simulink model "model2022b"  (R2022b)
settings: Solver=FixedStepAuto  StartTime=0.0  StopTime=25  FixedStep=0.01  RelTol=1e-3
undefined symbols (not defined in the file or in its folder): n1, n2
settings Model: Creator=Atread  LastModifiedBy=Atread
settings OptimizationCC: OptimizeBlockIOStorage=off  ReuseModelBlockBuffer=on  OptimizeDataStoreBuffers=off  BusAssignmentInplaceUpdate=off
settings DebuggingCC: SFUnexpectedBacktrackingDiag=warning  SFNoUnconditionalDefaultTransitionDiag=warning
settings RTWCC: GenerateReport=on  BuildConfiguration=Debug  LaunchReport=on  GPUComputeCapability=5.0
settings CodeAppCC: ForceParamTrailComments=on  MATLABSourceComments=on  EnableCustomComments=on
settings GRTTargetCC: CombineSignalStateStructs=on  SupportVariableSizeSignals=on  MultiInstanceErrorCode=Warning
settings ConfigComp: CovBoundaryAbsTol=1.0e-5

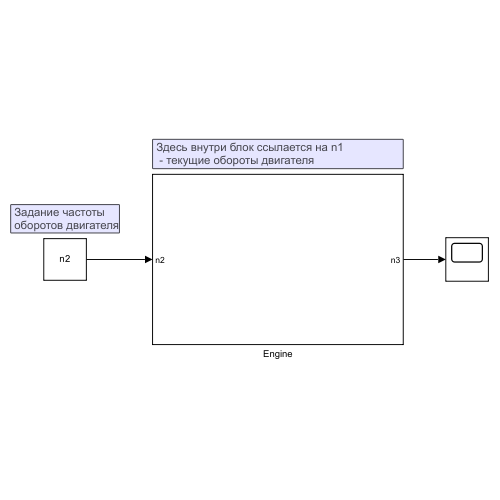
[thumbnail: Simulink's stored preview of the top-level diagram]
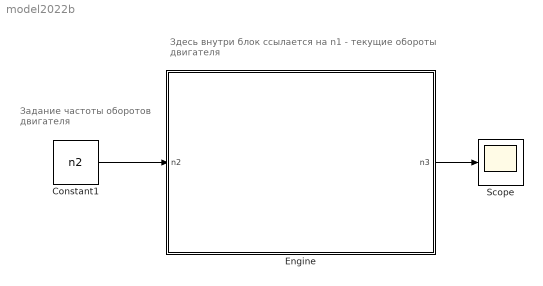
== system model2022b ==
  note: Здесь внутри блок ссылается на n1
      |  - текущие обороты двигателя
  note: Задание частоты
      | оборотов двигателя
  Constant1 : Constant  Value=n2
  Engine : Subsystem
  Scope : Scope
  wires:
  Constant1/1 -> Engine/1(n2)
  Engine/1(n3) -> Scope/1

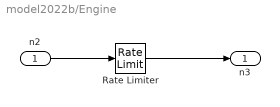
== system model2022b/Engine ==
  n2 : Inport
  Rate Limiter : RateLimiter  RisingSlewLimit=250  FallingSlewLimit=-250  SampleTimeMode=inherited  InitialCondition=n1
  n3 : Outport
  wires:
  n2/1 -> Rate Limiter/1
  Rate Limiter/1 -> n3/1
